simulink model "schema_simout"  (R2016a)
settings: Solver=FixedStepAuto  StartTime=0.0  StopTime=100  FixedStep=0.1  RelTol=1e-3
values from neighbouring files (symbols this model uses):
  A = [0 1; -0.2 -0.3]    [zis_seme_3.m]
  B = [0; 0.2]    [zis_seme_3.m]
  Bf = [0; 0.2]    [zis_seme_3.m]
  C = [1 0; 0 1]    [zis_seme_3.m]
  Df = [0; 1]    [zis_seme_3.m]
  K = (A + [1 0; 0 1])*inv(C)    [zis_seme_3.m]
settings Model: Creator=marek  LastModifiedBy=JK
settings GRTTargetCC: GeneratePreprocessorConditionals=Use local settings

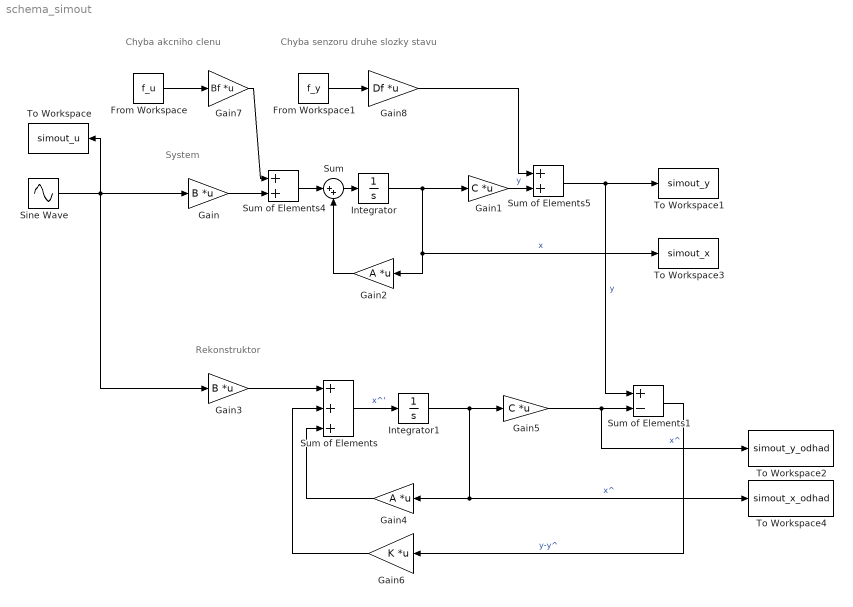
== system schema_simout ==
  note: Chyba senzoru
      | druhe slozky stavu
  note: Chyba akcniho clenu
  note: Rekonstruktor
  note: System
  From Workspace : FromWorkspace  VariableName=f_u  SampleTime=0
  From Workspace1 : FromWorkspace  VariableName=f_y  SampleTime=0
  Gain : Gain  Gain=B  Multiplication=Matrix(K*u)
  Gain1 : Gain  Gain=C  Multiplication=Matrix(K*u)
  Gain2 : Gain  Gain=A  Multiplication=Matrix(K*u)
  Gain3 : Gain  Gain=B  Multiplication=Matrix(K*u)
  Gain4 : Gain  Gain=A  Multiplication=Matrix(K*u)
  Gain5 : Gain  Gain=C  Multiplication=Matrix(K*u)
  Gain6 : Gain  Gain=K  Multiplication=Matrix(K*u)
  Gain7 : Gain  Gain=Bf  Multiplication=Matrix(K*u)
  Gain8 : Gain  Gain=Df  Multiplication=Matrix(K*u)
  Integrator : Integrator
  Integrator1 : Integrator
  Sine Wave : Sin  Amplitude=2  Frequency=0.2  Phase=0.3  SampleTime=0
  Sum : Sum  Inputs=|++
  Sum of Elements : Sum  Inputs=+++
  Sum of Elements1 : Sum  Inputs=+-
  Sum of Elements4 : Sum
  Sum of Elements5 : Sum
  To Workspace : ToWorkspace  VariableName=simout_u  SaveFormat=Timeseries  SampleTime=-1
  To Workspace1 : ToWorkspace  VariableName=simout_y  SaveFormat=Timeseries  SampleTime=-1
  To Workspace2 : ToWorkspace  VariableName=simout_y_odhad  SaveFormat=Timeseries  SampleTime=-1
  To Workspace3 : ToWorkspace  VariableName=simout_x  SaveFormat=Timeseries  SampleTime=-1
  To Workspace4 : ToWorkspace  VariableName=simout_x_odhad  SaveFormat=Timeseries  SampleTime=-1
  wires:
  Sine Wave/1 -> To Workspace/1, Gain3/1, Gain/1
  Sum/1 -> Integrator/1
  Integrator/1 -> To Workspace3/1, Gain2/1, Gain1/1  "x"
  Gain1/1 -> Sum of Elements5/2  "y"
  Gain2/1 -> Sum/2
  Gain3/1 -> Sum of Elements/1
  Sum of Elements/1 -> Integrator1/1  "x^'"
  Integrator1/1 -> To Workspace4/1, Gain4/1, Gain5/1  "x^"
  Gain5/1 -> To Workspace2/1, Sum of Elements1/2  "x^"
  Gain4/1 -> Sum of Elements/3
  Gain6/1 -> Sum of Elements/2
  Sum of Elements1/1 -> Gain6/1  "y-y^"
  Sum of Elements4/1 -> Sum/1
  Gain/1 -> Sum of Elements4/2
  From Workspace/1 -> Gain7/1
  Gain7/1 -> Sum of Elements4/1
  From Workspace1/1 -> Gain8/1
  Sum of Elements5/1 -> Sum of Elements1/1, To Workspace1/1  "y"
  Gain8/1 -> Sum of Elements5/1
